simulink model "HW1_MAE6280"  (Simulink 9.1)
settings: Solver=VariableStepAuto  StartTime=0.0  StopTime=10.0  RelTol=1e-3
InitFcn:
  | u0=0.01
libraries: simulink x1
settings Model: SuppressorTable=22 serialization::archive 11 0 6 0 0 0 0 0  Creator=hanfengzhai  LastModifiedBy=hanfengzhai
settings DataIOCC: SaveFormat=Dataset
settings OptimizationCC: LifeSpan=auto
settings DebuggingCC: UnderspecifiedInitializationDetection=Simplified  MergeDetectMultiDrivingBlocksExec=error  SFUnexpectedBacktrackingDiag=error  SFNoUnconditionalDefaultTransitionDiag=error  SFExecutionAtInitializationDiag=warning
settings HardwareCC: ProdBitPerPointer=64  ProdBitPerSizeT=64  ProdBitPerPtrDiffT=64  ProdLargestAtomicFloat=Float  ProdIntDivRoundTo=Zero  ProdEndianess=LittleEndian  ProdWordSize=64  ProdHWDeviceType=Intel->x86-64 (Windows64)
settings ModelReferenceCC: PropagateSignalLabelsOutOfModel=on
settings CodeAppCC: StateflowObjectComments=off
settings GRTTargetCC: TargetLangStandard=C99 (ISO)  CombineOutputUpdateFcns=on  GRTInterface=off
settings ConfigComp: CovMetricSettings=dwe  CovHtmlReporting=off  CovSaveCumulativeToWorkspaceVar=off  CovSaveSingleToWorkspaceVar=off  CovExternalEMLEnable=on

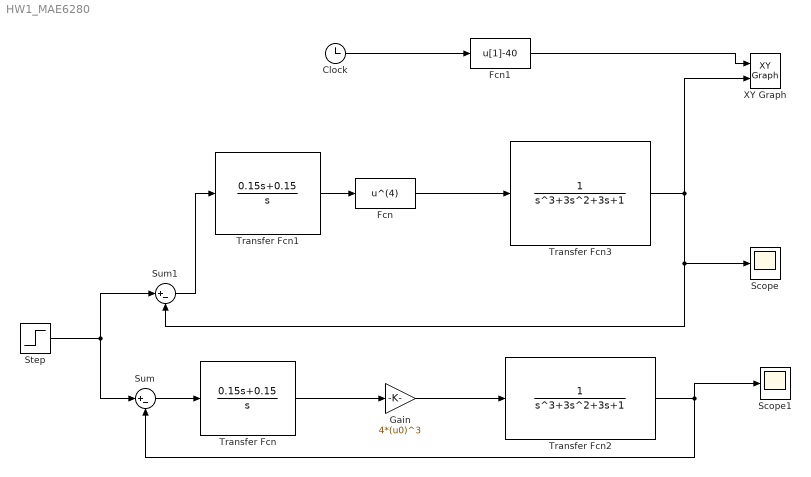
== system HW1_MAE6280 ==
  Clock : Clock
  Fcn : Fcn  Expr=u^(4)
  Fcn1 : Fcn  Expr=u[1]-40
  Gain : Gain  Gain=4*(u0)^3
  Scope : Scope
  Scope1 : Scope
  Step : Step  SampleTime=0
  Sum : Sum  Inputs=|+-
  Sum1 : Sum  Inputs=|+-
  Transfer Fcn : TransferFcn  Numerator=[0.15 0.15]  Denominator=[1 0]
  Transfer Fcn1 : TransferFcn  Numerator=[0.15 0.15]  Denominator=[1 0]
  Transfer Fcn2 : TransferFcn  Denominator=[1 3 3 1]
  Transfer Fcn3 : TransferFcn  Denominator=[1 3 3 1]
  XY Graph : simulink/Sinks/XY Graph  xmin=-1  xmax=1  ymin=-1  ymax=1  st=-1
  wires:
  Step/1 -> Sum/1, Sum1/1
  Sum/1 -> Transfer Fcn/1
  Clock/1 -> Fcn1/1
  Fcn1/1 -> XY Graph/1
  Transfer Fcn/1 -> Gain/1
  Sum1/1 -> Transfer Fcn1/1
  Transfer Fcn2/1 -> Scope1/1, Sum/2
  Transfer Fcn3/1 -> Sum1/2, Scope/1, XY Graph/2
  Transfer Fcn1/1 -> Fcn/1
  Fcn/1 -> Transfer Fcn3/1
  Gain/1 -> Transfer Fcn2/1
